simulink model "DistributedControllers"  (R2018b)
settings: Solver=ode1  StartTime=0.0  StopTime=10000  FixedStep=1  RelTol=1e-3
InitFcn:
  | clearvars
  | % Initializing FMIKit and adding paths
  | FMIKit.initialize
  | addpath('C:\Users\u375749\Documents\Thesis\Codes\Linearization')
  | addpath('C:\Users\u375749\Documents\Thesis\Codes\MatlabPlant')
  | % 'Running modelcreation_simplified.m
  | modelcreation_simplified
  | % Running substitution_simplified.m
  | [A,B,C,D] = constantsave(A,B,C,D,Qcont);
  | substitution_simplified
  | % Running kfinit_simulink.m
  | kfinit_simulink
  | % Running distributedControllers.m
  | distributedControllers
  | % Clear general variables
  | clear u
values from neighbouring files (symbols this model uses):
  delta_hValues = [0 114500]    [TGC.mat]
  initial =     [TGC.mat]
  kf = KalmanFilter    [kfinit_simulink.m]
  nu = 12    [TGC.mat]    (also in constants.mat = 11; constantsave.m = size(B,2))
  nx = 8    [TGC.mat]    (also in constants.mat = 9; constantsave.m = length(A))
  ny = 6    [TGC.mat]    (also in constants.mat; constantsave.m = size(C,1); estimatortest_simulink.m = size(Y,2))
  PI_C = PIController    [distributedControllers.m]
  PI_F = PIController    [distributedControllers.m]
  PI_GC = PIController    [distributedControllers.m]
  PI_HP = PIController    [distributedControllers.m]
  PI_LT = PIController    [distributedControllers.m]
  PI_MT = PIController    [distributedControllers.m]
  PI_RP = PIController    [distributedControllers.m]
  sigma = 6484.30967514    [TGC.mat]    (also in estimatortest.m = TauValues(4)/Ts*(DQ/DT - sigma)+ sigma; paramesttester.m = TauValues(4)/Ts*(DQ/DT - sigma)+ sigma; residualtest.m = DQ/DT)
  system =     [TGC.mat]
  Ts = 1    [LTVsystemDescription.m]    (also in TGC.mat; distributedControllers.m; kfinit_simulink.m)
undefined symbols (not defined in the file or in its folder): CoolProp, LTVsystemDescription, x2q
libraries: FMIKit_blocks x1
settings Model: Creator=U370698  LastModifiedBy=U375749
settings DebuggingCC: LibraryContextMissingDiagnostic=none  UnderSpecifiedDimensionMsg=warning
settings SFSimCC: SimUseLocalCustomCode=off
settings RTWCC: RTWUseLocalCustomCode=off

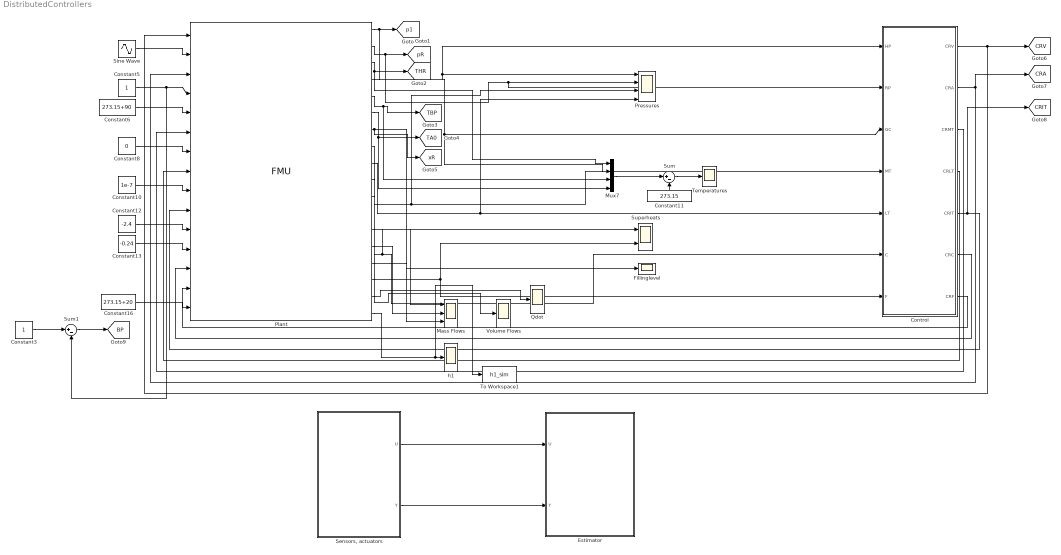
== system DistributedControllers ==
  Constant10 : Constant  Value=1e-7
  Constant11 : Constant  Value=273.15
  Constant12 : Constant  Value=-2.4
  Constant13 : Constant  Value=-0.24
  Constant16 : Constant  Value=273.15+20
  Constant3 : Constant
  Constant5 : Constant
  Constant6 : Constant  Value=273.15+90
  Constant8 : Constant  Value=0
  Control : Subsystem
  Estimator : Subsystem
  Fillinglevel : Scope
  Mass Flows : Scope  NumInputPorts=3
  Mux7 : Mux
  Plant : FMIKit_blocks/FMU  SFunctionModules=''
      settings: SourceProductName=FMI Kit
  Pressures : Scope  NumInputPorts=4
  Qdot : Scope
  "Sensors, actuators" : Subsystem
  Sine Wave : Sin  Amplitude=5  Bias=273.15+25  Frequency=2*pi*10/10000  Phase=pi/2  SampleTime=0
  Sum : Sum  Inputs=|+-
  Sum1 : Sum  Inputs=|+-
  Superheats : Scope  NumInputPorts=2
  Temperatures : Scope
  To Workspace1 : ToWorkspace  VariableName=h1_sim  SaveFormat=Structure With Time  SampleTime=-1
  Volume Flows : Scope
  h1 : Scope
  tag scope: BP=global, CRA=global, CRIT=global, CRV=global, TA0=global, TBP=global, THR=global, p1=global, pR=global, xR=global
  wires:
  Sine Wave/1 -> Plant/2
  Constant5/1 -> Sum1/2, Plant/4
  Constant6/1 -> Plant/5
  Constant8/1 -> Plant/7
  Constant10/1 -> Plant/9
  Constant12/1 -> Plant/11
  Constant13/1 -> Plant/12
  Constant16/1 -> Plant/15
  Plant/1 -> [p1], Pressures/1, Control/1(HP)
  Constant11/1 -> Sum/2
  Sum/1 -> Temperatures/1
  Mux7/1 -> Sum/1
  Plant/3 -> [THR], Mux7/1
  Control/1(CRV) -> [CRV], Plant/1
  Control/2(CRA) -> [CRA], Plant/3
  Control/3(CRMT) -> Plant/6
  Control/4(CRLT) -> Plant/8
  Control/6(CRC) -> Plant/13
  Control/7(CRF) -> Plant/14
  Plant/11 -> Control/7(F), Superheats/2
  Plant/10 -> Superheats/1, Control/6(C)
  Plant/9 -> Pressures/4, Control/5(LT)
  Plant/8 -> Pressures/3, Control/4(MT)
  Plant/7 -> [xR], Fillinglevel/1
  Plant/6 -> [TA0], Mux7/4
  Plant/4 -> Control/3(GC), Mux7/2
  Plant/5 -> [TBP], Mux7/3
  Constant3/1 -> Sum1/1
  Sum1/1 -> [BP]
  Plant/2 -> [pR], Control/2(RP), Pressures/2
  Plant/13 -> Mass Flows/1
  Plant/14 -> Mass Flows/2
  Plant/15 -> Mass Flows/3
  Plant/16 -> Volume Flows/1
  Plant/17 -> Qdot/1
  Plant/18 -> To Workspace1/1, h1/1
  Control/5(CRIT) -> [CRIT], Plant/10
  "Sensors, actuators"/1(U) -> Estimator/1(U)
  "Sensors, actuators"/2(Y) -> Estimator/2(Y)

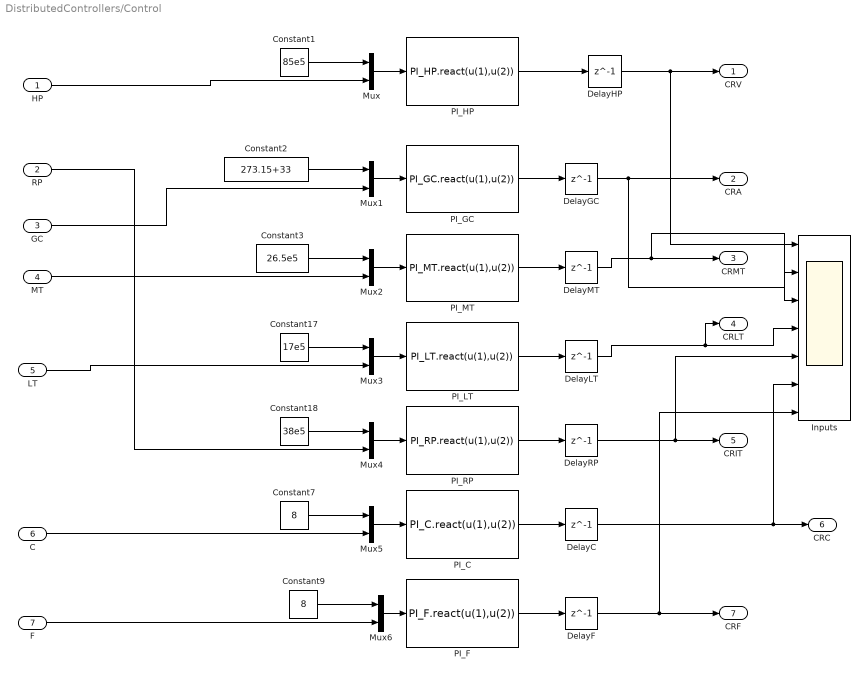
== system DistributedControllers/Control ==
  HP : Inport
  RP : Inport  Port=2
  GC : Inport  Port=3
  MT : Inport  Port=4
  LT : Inport  Port=5
  C : Inport  Port=6
  F : Inport  Port=7
  Constant1 : Constant  Value=85e5
  Constant17 : Constant  Value=17e5
  Constant18 : Constant  Value=38e5
  Constant2 : Constant  Value=273.15+33
  Constant3 : Constant  Value=26.5e5
  Constant7 : Constant  Value=8
  Constant9 : Constant  Value=8
  DelayC : Delay  DelayLength=1  InitialCondition=0.1
  DelayF : Delay  DelayLength=1  InitialCondition=0.04
  DelayGC : Delay  DelayLength=1  InitialCondition=0.625
  DelayHP : Delay  DelayLength=1  InitialCondition=0.25
  DelayLT : Delay  DelayLength=1  InitialCondition=0.3
  DelayMT : Delay  DelayLength=1  InitialCondition=0.3
  DelayRP : Delay  DelayLength=1  InitialCondition=0.45
  Inputs : Scope  NumInputPorts=7
  Mux{,1..6} (7 alike) : Mux  Inputs=2
  PI_C : MATLABFcn  MATLABFcn=PI_C.react(u(1),u(2))
  PI_F : MATLABFcn  MATLABFcn=PI_F.react(u(1),u(2))
  PI_GC : MATLABFcn  MATLABFcn=PI_GC.react(u(1),u(2))
  PI_HP : MATLABFcn  MATLABFcn=PI_HP.react(u(1),u(2))
  PI_LT : MATLABFcn  MATLABFcn=PI_LT.react(u(1),u(2))
  PI_MT : MATLABFcn  MATLABFcn=PI_MT.react(u(1),u(2))
  PI_RP : MATLABFcn  MATLABFcn=PI_RP.react(u(1),u(2))
  CRV : Outport
  CRA : Outport  Port=2
  CRMT : Outport  Port=3
  CRLT : Outport  Port=4
  CRIT : Outport  Port=5
  CRC : Outport  Port=6
  CRF : Outport  Port=7
  wires:
  MT/1 -> Mux2/2
  Mux3/1 -> PI_LT/1
  Mux4/1 -> PI_RP/1
  DelayHP/1 -> Inputs/1, CRV/1
  Mux1/1 -> PI_GC/1
  DelayLT/1 -> Inputs/4, CRLT/1
  Constant2/1 -> Mux1/1
  Mux6/1 -> PI_F/1
  PI_HP/1 -> DelayHP/1
  Constant1/1 -> Mux/1
  PI_MT/1 -> DelayMT/1
  PI_LT/1 -> DelayLT/1
  PI_GC/1 -> DelayGC/1
  Mux2/1 -> PI_MT/1
  Constant18/1 -> Mux4/1
  Mux5/1 -> PI_C/1
  Constant7/1 -> Mux5/1
  Constant3/1 -> Mux2/1
  Constant9/1 -> Mux6/1
  PI_C/1 -> DelayC/1
  PI_F/1 -> DelayF/1
  PI_RP/1 -> DelayRP/1
  F/1 -> Mux6/2
  HP/1 -> Mux/2
  Constant17/1 -> Mux3/1
  Mux/1 -> PI_HP/1
  GC/1 -> Mux1/2
  LT/1 -> Mux3/2
  DelayRP/1 -> Inputs/5, CRIT/1
  DelayC/1 -> CRC/1, Inputs/6
  DelayF/1 -> Inputs/7, CRF/1
  C/1 -> Mux5/2
  DelayGC/1 -> Inputs/2, CRA/1
  RP/1 -> Mux4/2
  DelayMT/1 -> Inputs/3, CRMT/1

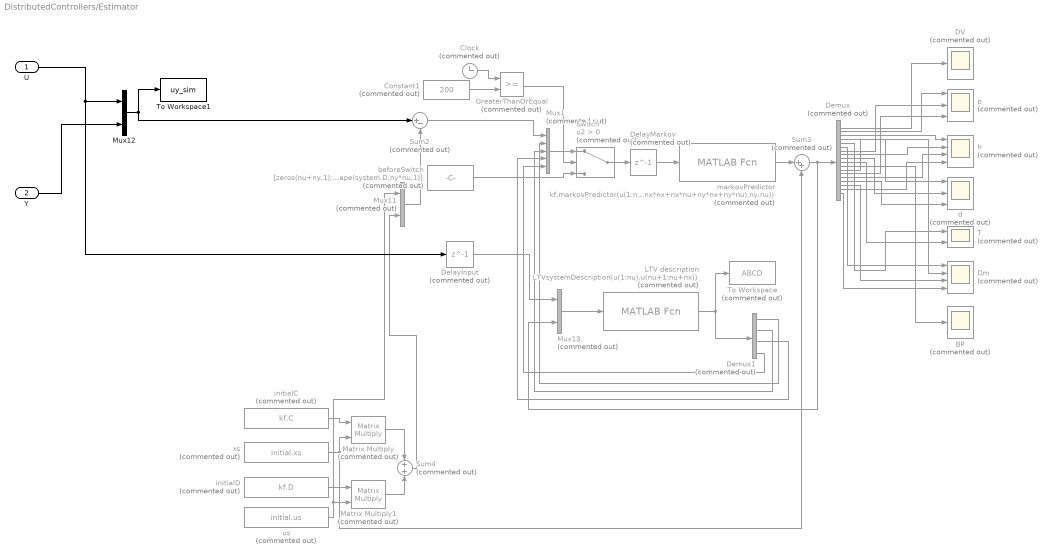
== system DistributedControllers/Estimator ==
  U : Inport
  Y : Inport  Port=2
  BP : Scope  Commented=on
  Clock : Clock  Commented=on
  Constant1 : Constant  Commented=on  Value=200
  DV : Scope  Commented=on
  DelayInput : Delay  Commented=on  DelayLength=1  InitialCondition=[initial.us]
  DelayMarkov : Delay  Commented=on  DelayLength=1  InitialCondition=[zeros(nu+ny,1); reshape(system.A,nx*nx,1); reshape(system.B,nx*nu,1); reshape(system.C,ny*nx,1); reshape(system.D,ny*nu,1)]
  Demux : Demux  Commented=on  Outputs=18
  Demux1 : Demux  Commented=on  Outputs=[nx*nx; nx*nu; ny*nx; ny*nu]
  Dm : Scope  Commented=on  NumInputPorts=4
  GreaterThanOrEqual : RelationalOperator  Commented=on  OutDataTypeStr=boolean  RndMeth=Simplest
  LTV description : MATLABFcn  Commented=on  MATLABFcn=LTVsystemDescription(u(1:nu),u(nu+1:nu+nx))
  Matrix Multiply : Product  Commented=on  Multiplication=Matrix(*)
  Matrix Multiply1 : Product  Commented=on  Multiplication=Matrix(*)
  Mux1 : Mux  Commented=on  Inputs=5
  Mux11 : Mux  Commented=on  Inputs=2
  Mux12 : Mux  Inputs=2
  Mux13 : Mux  Commented=on  Inputs=2
  Sum2 : Sum  Commented=on  Inputs=|+-
  Sum3 : Sum  Commented=on  Inputs=|++
  Sum4 : Sum  Commented=on  Inputs=+|+
  Switch : Switch  Commented=on  Criteria=u2 > Threshold
  T : Scope  Commented=on  NumInputPorts=2
  To Workspace : ToWorkspace  Commented=on  VariableName=ABCD  SaveFormat=Structure With Time  SampleTime=-1
  To Workspace1 : ToWorkspace  VariableName=uy_sim  SaveFormat=Structure With Time  SampleTime=-1
  beforeSwitch : Constant  Commented=on  Value=[zeros(nu+ny,1); reshape(system.A,nx*nx,1); reshape(system.B,nx*nu,1); reshape(system.C,ny*nx,1); reshape(system.D,ny*nu,1)]
  d : Scope  Commented=on  NumInputPorts=3
  h : Scope  Commented=on  NumInputPorts=4
  initialC : Constant  Commented=on  Value=kf.C
  initialD : Constant  Commented=on  Value=kf.D
  markovPredictor : MATLABFcn  Commented=on  MATLABFcn=kf.markovPredictor(u(1:nu),u(nu+1:nu+ny),reshape(u(nu+ny+1:nu+ny+nx*nx),nx,nx),reshape(u(nu+ny+nx*nx+1:nu+ny+nx*nx+nx*nu),nx,nu),reshape(u(nu+ny+nx*nx+nx*nu+1:nu+ny+nx*nx+nx*nu+ny*nx),ny,nx), reshape(u(nu+ny+nx*nx+nx*nu+ny*nx+1:nu+ny+nx*nx+nx*nu+ny*nx+ny*nu),ny,nu))
  p : Scope  Commented=on  NumInputPorts=3
  us : Constant  Commented=on  Value=initial.us
  xs : Constant  Commented=on  Value=initial.xs
  wires:
  Demux/1 -> DV/1
  Demux/17 -> h/4
  Demux/9 -> d/2
  Demux1/4 -> Mux1/5
  Mux12/1 -> Sum2/1, To Workspace1/1
  Matrix Multiply/1 -> Sum4/1
  xs/1 -> Sum3/2, Matrix Multiply/2
  Demux/15 -> d/3
  Demux/13 -> p/3
  Demux/7 -> p/2
  Demux/10 -> T/2
  Demux/8 -> h/2
  Demux/5 -> T/1
  Demux/14 -> h/3
  Clock/1 -> GreaterThanOrEqual/1
  initialD/1 -> Matrix Multiply1/1
  Demux/2 -> p/1
  initialC/1 -> Matrix Multiply/1
  Mux11/1 -> Sum2/2
  Demux/18 -> Dm/4
  Demux/12 -> Dm/2
  Y/1 -> Mux12/2
  beforeSwitch/1 -> Switch/3
  Constant1/1 -> GreaterThanOrEqual/2
  GreaterThanOrEqual/1 -> Switch/2
  Demux/16 -> Dm/3
  Demux/11 -> BP/1
  us/1 -> Matrix Multiply1/2, Mux11/1
  markovPredictor/1 -> Sum3/1
  Sum2/1 -> Mux1/1
  DelayMarkov/1 -> markovPredictor/1
  Demux1/2 -> Mux1/3
  Sum4/1 -> Mux11/2
  Demux1/1 -> Mux1/2
  LTV description/1 -> Demux1/1, To Workspace/1
  Mux1/1 -> Switch/1
  Demux/3 -> h/1
  U/1 -> DelayInput/1, Mux12/1
  Mux13/1 -> LTV description/1
  Matrix Multiply1/1 -> Sum4/2
  Demux1/3 -> Mux1/4
  Switch/1 -> DelayMarkov/1
  Sum3/1 -> Mux13/2, Demux/1
  DelayInput/1 -> Mux13/1
  Demux/6 -> Dm/1
  Demux/4 -> d/1

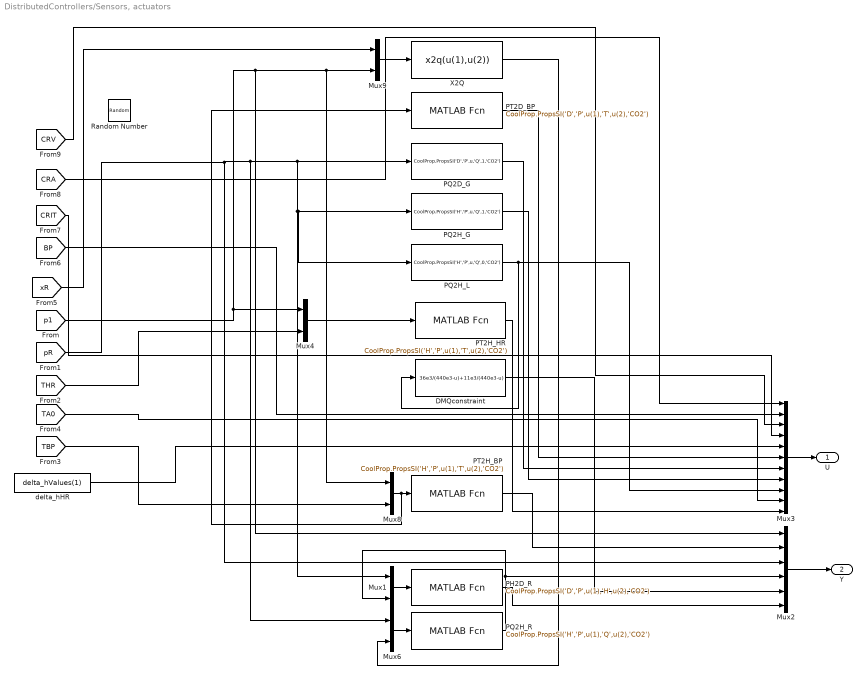
== system DistributedControllers/Sensors, actuators ==
  DMQconstraint : MATLABFcn  MATLABFcn=36e3/(440e3-u)+11e3/(440e3-u)
  Mux{1,4,6,8..9} (5 alike) : Mux  Inputs=2
  Mux2 : Mux  Inputs=6
  Mux3 : Mux  Inputs=11
  PH2D_R : MATLABFcn  MATLABFcn=CoolProp.PropsSI('D','P',u(1),'H',u(2),'CO2')
  PQ2D_G : MATLABFcn  MATLABFcn=CoolProp.PropsSI('D','P',u,'Q',1,'CO2')
  PQ2H_G : MATLABFcn  MATLABFcn=CoolProp.PropsSI('H','P',u,'Q',1,'CO2')
  PQ2H_L : MATLABFcn  MATLABFcn=CoolProp.PropsSI('H','P',u,'Q',0,'CO2')
  PQ2H_R : MATLABFcn  MATLABFcn=CoolProp.PropsSI('H','P',u(1),'Q',u(2),'CO2')
  PT2D_BP : MATLABFcn  MATLABFcn=CoolProp.PropsSI('D','P',u(1),'T',u(2),'CO2')
  PT2H_BP : MATLABFcn  MATLABFcn=CoolProp.PropsSI('H','P',u(1),'T',u(2),'CO2')
  PT2H_HR : MATLABFcn  MATLABFcn=CoolProp.PropsSI('H','P',u(1),'T',u(2),'CO2')
  Random Number : RandomNumber  Variance=sigma/Ts  SampleTime=0.1
  X2Q : MATLABFcn  MATLABFcn=x2q(u(1),u(2))
  delta_hHR : Constant  Value=delta_hValues(1)
  U : Outport
  Y : Outport  Port=2
  wires:
  [pR] -> Mux6/1, Mux1/1, PQ2H_L/1, PQ2H_G/1, PQ2D_G/1, Mux2/3
  PT2H_HR/1 -> Mux3/11
  [p1] -> Mux2/1, Mux8/1, Mux9/2, Mux4/1
  PQ2H_L/1 -> Mux3/9, DMQconstraint/1
  [TBP] -> Mux8/2
  [xR] -> Mux9/1
  [CRIT] -> Mux3/4
  PQ2H_R/1 -> Mux1/2, Mux2/4
  PT2D_BP/1 -> Mux3/6
  [TA0] -> Mux3/10
  [THR] -> Mux4/2
  PH2D_R/1 -> Mux2/6
  [BP] -> Mux3/2
  DMQconstraint/1 -> Mux2/5
  Mux9/1 -> X2Q/1
  [CRV] -> Mux3/3
  [CRA] -> Mux3/1
  PT2H_BP/1 -> Mux2/2
  PQ2D_G/1 -> Mux3/7
  Mux8/1 -> PT2D_BP/1, PT2H_BP/1
  Mux4/1 -> PT2H_HR/1
  X2Q/1 -> Mux6/2
  PQ2H_G/1 -> Mux3/8
  Mux6/1 -> PQ2H_R/1
  delta_hHR/1 -> Mux3/5
  Mux1/1 -> PH2D_R/1
  Mux3/1 -> U/1
  Mux2/1 -> Y/1
